simulink model "Isooffboard_SSC"  (R2025b)
settings: Solver=VariableStepAuto  StartTime=0.0  StopTime=0.5  RelTol=1e-3
undefined symbols (not defined in the file): V_ref_isolated
libraries: fl_lib x73, nesl_utility x29, ee_lib x9, simulink x3, eeTransforms x2, batteryecm_lib x1, eeSinusoidalMeasurementV2 x1
(part 3 of 3)

== matlab function Isooffboard_SSC/Subsystem7/MATLAB Function ==
  data: u input; y output
function y = fcn(u)
persistent t;
if isempty (t)
t=0;
end
frequency = u*105310; %105310 
t=t+0.0000001;

y = (sawtooth(2 * pi * frequency * t, 0.5)+1)/2;
